simulink model "TransmissionMode_plausibility"  (R2024b)
settings: Solver=FixedStepAuto  StartTime=0.0  StopTime=20  RelTol=1e-3
settings Model: Creator=aayan  LastModifiedBy=aayan
settings ConfigComp: CovEnable=on  RecordCoverage=on  CovMetricSettings=dcmwe  CovModelRefEnable=on

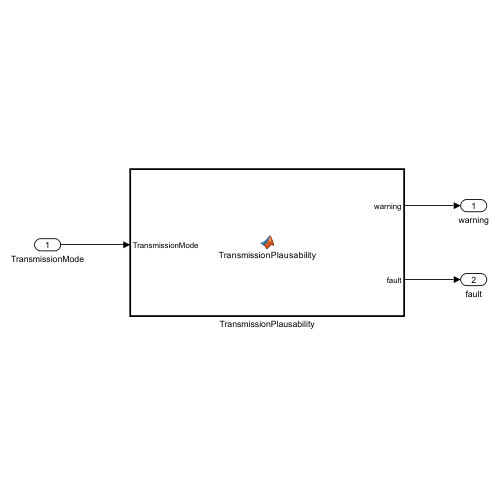
[thumbnail: Simulink's stored preview of the top-level diagram]
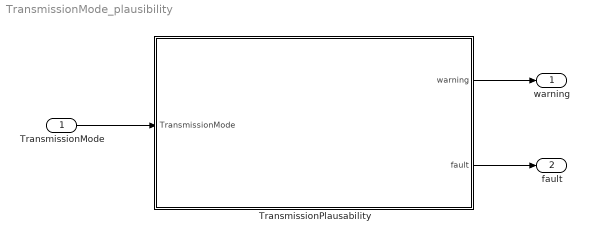
== system TransmissionMode_plausibility ==
  TransmissionMode : Inport  OutDataTypeStr=Enum: TransmissionState
  TransmissionPlausability : MATLAB Function  TreatAsAtomicUnit=on
  warning : Outport
  fault : Outport  Port=2
  wires:
  TransmissionPlausability/1(warning) -> warning/1
  TransmissionPlausability/2(fault) -> fault/1
  TransmissionMode/1 -> TransmissionPlausability/1(TransmissionMode)

== matlab function TransmissionMode_plausibility/TransmissionPlausability ==
  data: TransmissionMode input; warning output; fault output
function [warning, fault] = TransmissionPlausability(TransmissionMode)

% initialization
warning = boolean(0);
fault = boolean(0);

validModes = [ ...
    TransmissionState.Park, ...
    TransmissionState.Reverse, ...
    TransmissionState.Neutral, ...
    TransmissionState.Drive, ...
    TransmissionState.Brake ...
];

if ~any(TransmissionMode == validModes)
    warning = boolean(1);
    fault = boolean(1);
end
